simulink model "ModelWodyKaskadowej"  (Simulink 8.0)
settings: Solver=ode45  SolverMode=SingleTasking  StartTime=0.0  StopTime=10.0  RelTol=1e-3
values from neighbouring files (symbols this model uses):
  A1 = 1    [Lab06.m]
  A2 = 2    [Lab06.m]
  Aw1 = 0.1.*A1    [Lab06.m]
  Aw2 = 0.1.*A2    [Lab06.m]
  fwe1 = 0.2.*fwe1max    [Lab06.m]
  g = 10    [Lab06.m]
undefined symbols (not defined in the file or in its folder): h10, h20
settings Model: Creator=jakub  LastModifiedBy=luki9  CovMetricSettings=dwe  CovHtmlReporting=off  covSaveCumulativeToWorkspaceVar=off  CovSaveSingleToWorkspaceVar=off  CovExternalEMLEnable=on
settings DataIOCC: LimitDataPoints=off  SaveFormat=StructureWithTime  ReturnWorkspaceOutputs=on
settings OptimizationCC: ExpressionDepthLimit=128
settings DebuggingCC: UnderspecifiedInitializationDetection=Simplified  MergeDetectMultiDrivingBlocksExec=error  SolverPrmCheckMsg=none  FrameProcessingCompatibilityMsg=error  StateNameClashWarn=none  SFUnexpectedBacktrackingDiag=error  SFNoUnconditionalDefaultTransitionDiag=error
settings HardwareCC: ProdBitPerPointer=64  ProdLargestAtomicFloat=Float  ProdIntDivRoundTo=Zero  ProdEndianess=LittleEndian  ProdHWDeviceType=Specified
settings ModelReferenceCC: PropagateSignalLabelsOutOfModel=on
settings SFSimCC: SimUseLocalCustomCode=on
settings RTWCC: RTWUseLocalCustomCode=on
settings CodeAppCC: CustomSymbolStrType=$N$R$M_T
settings GRTTargetCC: CodeReplacementLibrary=C99 (ISO)  GeneratePreprocessorConditionals=Use local settings

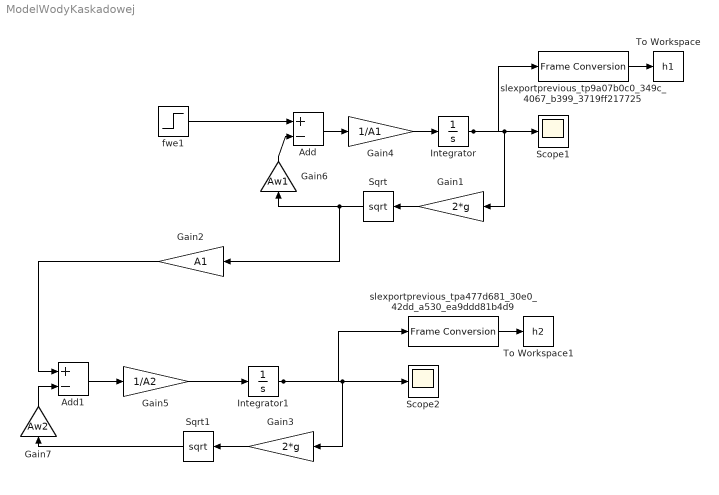
== system ModelWodyKaskadowej ==
  Add : Sum  Inputs=+-
  Add1 : Sum  Inputs=+-
  Gain1 : Gain  Gain=2*g
  Gain2 : Gain  Gain=A1
  Gain3 : Gain  Gain=2*g
  Gain4 : Gain  Gain=1/A1
  Gain5 : Gain  Gain=1/A2
  Gain6 : Gain  Gain=Aw1
  Gain7 : Gain  Gain=Aw2
  Integrator : Integrator  InitialCondition=h10
  Integrator1 : Integrator  InitialCondition=h20
  Scope1 : Scope
      settings: TimeRange=auto  MaxDataPoints=5000  SaveToWorkspace=off  YMin=1373.87947  YMax=1575.1245  SampleTime=-1
  Scope2 : Scope
      settings: TimeRange=auto  MaxDataPoints=5000  SaveToWorkspace=off  SaveName=ScopeData  YMin=1394.43662  YMax=3000.07045  SampleTime=-1
  Sqrt : Sqrt  SaturateOnIntegerOverflow=on
  Sqrt1 : Sqrt  SaturateOnIntegerOverflow=on
  To Workspace : ToWorkspace  VariableName=h1  SampleTime=-1
  To Workspace1 : ToWorkspace  VariableName=h2  SampleTime=-1
  "fwe1 " : Step  After=fwe1  SampleTime=0
  slexportprevious_tp9a07b0c0_349c_4067_b399_3719ff217725 : FrameConversion  OutFrame=Sample-based
  slexportprevious_tpa477d681_30e0_42dd_a530_ea9ddd81b4d9 : FrameConversion  OutFrame=Sample-based
  wires:
  "fwe1 "/1 -> Add/1
  Gain1/1 -> Sqrt/1
  Add/1 -> Gain4/1
  Integrator/1 -> Scope1/1, Gain1/1, slexportprevious_tp9a07b0c0_349c_4067_b399_3719ff217725/1
  Sqrt/1 -> Gain2/1, Gain6/1
  Add1/1 -> Gain5/1
  Integrator1/1 -> Scope2/1, Gain3/1, slexportprevious_tpa477d681_30e0_42dd_a530_ea9ddd81b4d9/1
  Gain3/1 -> Sqrt1/1
  Sqrt1/1 -> Gain7/1
  Gain4/1 -> Integrator/1
  Gain5/1 -> Integrator1/1
  Gain6/1 -> Add/2
  Gain7/1 -> Add1/2
  Gain2/1 -> Add1/1
  slexportprevious_tp9a07b0c0_349c_4067_b399_3719ff217725/1 -> To Workspace/1
  slexportprevious_tpa477d681_30e0_42dd_a530_ea9ddd81b4d9/1 -> To Workspace1/1
